simulink model "testro"  (Simulink 5.0)
settings: Solver=ode5  SolverMode=SingleTasking  StartTime=0.0  StopTime=inf  FixedStep=0.001  RelTol=1e-3
libraries: pci1711 x3, simulink_extras x2
settings Model: LastModifiedBy=AD  SimulationMode=external  RTWOptions="-aEnforceIntegerDowncast=1 -aExtMode=0 -aExtModeTesting=0 -aFoldNonRolledExpr=1 -aForceParamTrailComments=0 -aGenerateComments=1 -aGenerateReport=0 -aIgnoreCustomStorageClasses=1 -aIncDataTypeInIds=0 -aIncHierarchyInIds=0 -aInlineInvariantSignals=1 -aInlineParameters=0 -aInlinedPrmAccess=\"Literals\" -aLocalBlockOutputs=1 -aLogVarNameModifier=\"rt_\" -aMaxRTWIdLen=31 -aPrefixModelToSubsysFcnNames=1 -aRTWVerbose=1 -aRollThreshold=5 -aShowEliminatedStatements=0"

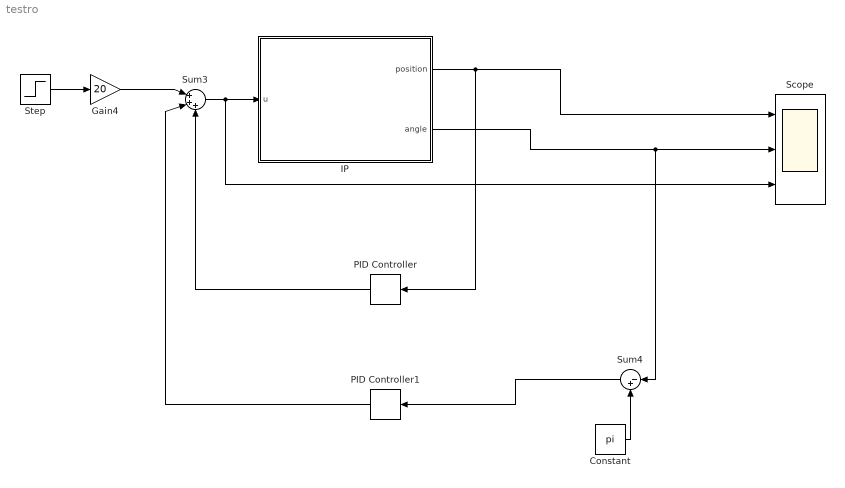
== system testro ==
  Constant : Constant  Value=pi
  Gain4 : Gain  Gain=20  SaturateOnIntegerOverflow=on
  IP : Subsystem
  PID Controller : simulink_extras/Additional Linear/PID Controller  Orientation=left  P=-31*2  I=0  D=-110
  PID Controller1 : simulink_extras/Additional Linear/PID Controller  Orientation=left  P=-25  I=0  D=-28
  Scope : Scope  NumInputPorts=3
      settings: TickLabels=on  TimeRange=50  YMin=-0.05~2.95~-150  YMax=0.35~3.4~125  Decimation=10  SampleInput=on  SampleTime=0.01
  Step : Step  Time=5  After=0.2  SampleTime=0
  Sum3 : Sum  Inputs=|+++  SaturateOnIntegerOverflow=on
  Sum4 : Sum  Orientation=left  Inputs=|-+  SaturateOnIntegerOverflow=on
  wires:
  IP/1(position) -> PID Controller/1, Scope/1
  IP/2(angle) -> Sum4/1, Scope/2
  Sum3/1 -> Scope/3, IP/1(u)
  Gain4/1 -> Sum3/1
  Step/1 -> Gain4/1
  PID Controller/1 -> Sum3/3
  PID Controller1/1 -> Sum3/2
  Constant/1 -> Sum4/2
  Sum4/1 -> PID Controller1/1

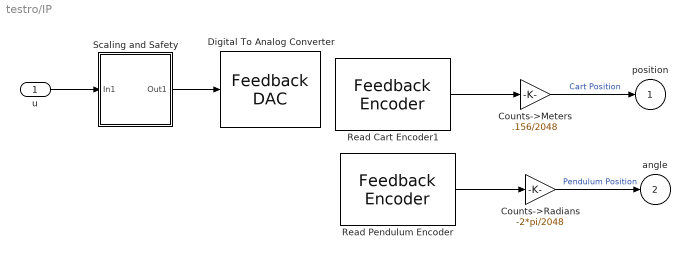
== system testro/IP ==
  u : Inport
  Counts->Meters : Gain  Gain=.156/2048  SaturateOnIntegerOverflow=on
  Counts->Radians : Gain  Gain=-2*pi/2048  SaturateOnIntegerOverflow=on
  Digital To Analog Converter : pci1711/Advantech  PCI1711 I//O Board Lib/Feedback DAC  channel=0  range=0  tsamp=0.001  hwAccess=on
  Read Cart Encoder1 : pci1711/Advantech  PCI1711 I//O Board Lib/Feedback Encoder   channel=0  offset=0  tsamp=0.001  hwAccess=on
  Read Pendulum Encoder : pci1711/Advantech  PCI1711 I//O Board Lib/Feedback Encoder   channel=1  offset=-1024  tsamp=0.001  hwAccess=on
  Scaling and Safety : Subsystem
  position : Outport
  angle : Outport  Port=2
  wires:
  Scaling and Safety/1(Out1) -> Digital To Analog Converter/1
  u/1 -> Scaling and Safety/1(In1)
  Read Cart Encoder1/1 -> Counts->Meters/1
  Read Pendulum Encoder/1 -> Counts->Radians/1
  Counts->Radians/1 -> angle/1  "Pendulum Position"
  Counts->Meters/1 -> position/1  "Cart Position"

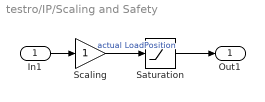
== system testro/IP/Scaling and Safety ==
  In1 : Inport
  Saturation : Saturate  UpperLimit=2.5  LowerLimit=-2.5
  Scaling : Gain  SaturateOnIntegerOverflow=on
  Out1 : Outport
  wires:
  Scaling/1 -> Saturation/1  "actual LoadPosition"
  In1/1 -> Scaling/1
  Saturation/1 -> Out1/1
